simulink model "Model_10_2"  (R2018a)
settings: Solver=VariableStepAuto  StartTime=0.0  StopTime=10.0  RelTol=1e-3
values from neighbouring files (symbols this model uses):
  bias_u = 0.2    [CEE_10.m]    (also in CEE_10_unc.m; CEE_11.m)
  C_I = [1 0 0 0 0]    [CEE_10.m]    (also in CEE_10_performance.m; CEE_11.m)
  covProcess = 100*diag([0.018^2,(0.018*10)^2,0.018^2,(0.018*10)^2,0.025^2])    [CEE_10.m]    (also in CEE_10_performance.m; CEE_10_unc.m; CEE_11.m; CEE_9.m)
  covSensor = ((0.018)^2)*eye(2)    [CEE_10.m]    (also in CEE_10_performance.m = ((2*0.018)^2)*eye(2); CEE_10_unc.m = ((2*0.018)^2)*eye(2); CEE_11.m; CEE_9.m)
  deadzone_u = 2e-1    (= 0.2)    [CEE_10.m]    (also in CEE_10_performance.m; CEE_10_unc.m; CEE_11.m; CEE_9.m = 0.1)
  L = lqe(A, G, C, Qe, Re)    [CEE_10.m]    (also in CEE_10_performance.m; CEE_10_unc.m; CEE_11.m; CEE_9.m)
  pulse = 4    [CEE_10.m]    (also in CEE_10_performance.m; CEE_10_unc.m; CEE_9.m; CEE_9_performance.m)
  saturation_u = 5    [CEE_10.m]    (also in CEE_10_performance.m; CEE_10_unc.m; CEE_11.m; CEE_9.m)
  tc = (1/100)*2*pi/10    (= 0.00628318530718)    [CEE_10.m]    (also in CEE_10_performance.m; CEE_10_unc.m; CEE_11.m; CEE_9.m)
  x0 = [50,0,10,0,0]'*pi/180    [CEE_10.m]    (also in CEE_10_performance.m; CEE_11.m; CEE_9.m; CEE_9_performance.m)
undefined symbols (not defined in the file or in its folder): A, B, C, K
libraries: simulink x2
settings Model: Creator=miguelsilva  LastModifiedBy=leonardopedroso
settings DebuggingCC: LibraryContextMissingDiagnostic=warning
settings SFSimCC: SimUseLocalCustomCode=on
settings RTWCC: RTWUseLocalCustomCode=on

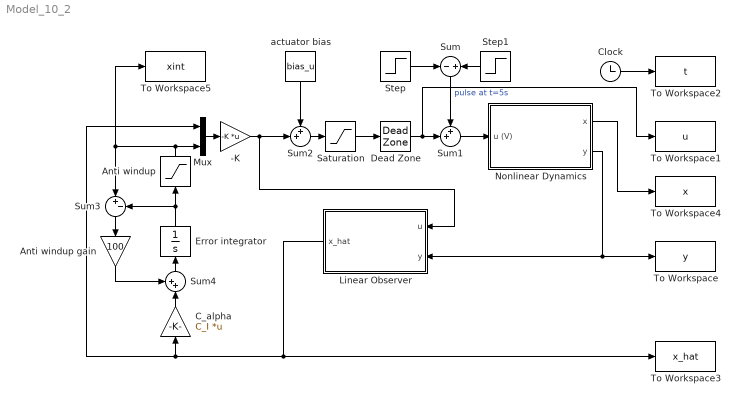
== system Model_10_2 ==
  -K : Gain  Gain=-K  Multiplication=Matrix(K*u) (u vector)
  Anti windup : Saturate  UpperLimit=0.3  LowerLimit=-0.3
  Anti windup gain : Gain  Gain=100
  C_alpha : Gain  Gain=C_I  Multiplication=Matrix(K*u) (u vector)
  Clock : Clock
  "Dead Zone " : DeadZone  LowerValue=-deadzone_u  UpperValue=deadzone_u  SaturateOnIntegerOverflow=on
  Error integrator : Integrator
  "Linear Observer " : Subsystem
  Mux : Mux  Inputs=2
  Nonlinear Dynamics : Subsystem
  "Saturation " : Saturate  UpperLimit=saturation_u  LowerLimit=-saturation_u
  Step : Step  Time=5.1  After=pulse  SampleTime=0
  Step1 : Step  Time=5  After=pulse  SampleTime=0
  Sum : Sum  Inputs=-|+
  Sum1 : Sum  Inputs=++|
  Sum2 : Sum  Inputs=++|
  Sum3 : Sum  Inputs=|+-
  Sum4 : Sum  Inputs=++|
  To Workspace : ToWorkspace  VariableName=y  SampleTime=-1
  To Workspace1 : ToWorkspace  VariableName=u  SampleTime=-1
  To Workspace2 : ToWorkspace  VariableName=t  SampleTime=-1
  To Workspace3 : ToWorkspace  VariableName=x_hat  SampleTime=-1
  To Workspace4 : ToWorkspace  VariableName=x  SampleTime=-1
  To Workspace5 : ToWorkspace  VariableName=xint  SampleTime=-1
  actuator bias : Constant  Value=bias_u
  wires:
  Clock/1 -> To Workspace2/1
  Nonlinear Dynamics/2(y) -> To Workspace/1, "Linear Observer "/2("y ")
  "Linear Observer "/1(x_hat) -> To Workspace3/1, C_alpha/1, Mux/1
  "Saturation "/1 -> "Dead Zone "/1
  Step/1 -> Sum/1
  Step1/1 -> Sum/2
  "Dead Zone "/1 -> To Workspace1/1, Sum1/2
  Sum1/1 -> Nonlinear Dynamics/1(u (V))
  Sum/1 -> Sum1/1  "pulse at t=5s"
  Nonlinear Dynamics/1(x) -> To Workspace4/1
  Mux/1 -> -K/1
  -K/1 -> Sum2/2, "Linear Observer "/1(u)
  Sum2/1 -> "Saturation "/1
  actuator bias/1 -> Sum2/1
  Anti windup/1 -> Sum3/1, To Workspace5/1, Mux/2
  Error integrator/1 -> Sum3/2, Anti windup/1
  Sum4/1 -> Error integrator/1
  C_alpha/1 -> Sum4/2
  Sum3/1 -> Anti windup gain/1
  Anti windup gain/1 -> Sum4/1

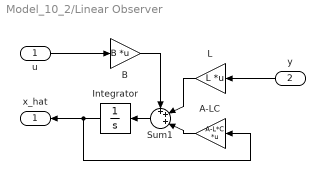
== system Model_10_2/Linear Observer  ==
  u : Inport
  "y " : Inport  Port=2
  A-LC : Gain  Gain=A-L*C  Multiplication=Matrix(K*u) (u vector)
  B : Gain  Gain=B  Multiplication=Matrix(K*u) (u vector)
  Integrator : Integrator  InitialCondition=zeros(5,1)
  L : Gain  Gain=L  Multiplication=Matrix(K*u) (u vector)
  Sum1 : Sum  Inputs=+++|
  x_hat : Outport
  wires:
  Integrator/1 -> x_hat/1, A-LC/1
  L/1 -> Sum1/2
  "y "/1 -> L/1
  Sum1/1 -> Integrator/1
  A-LC/1 -> Sum1/3
  B/1 -> Sum1/1
  u/1 -> B/1

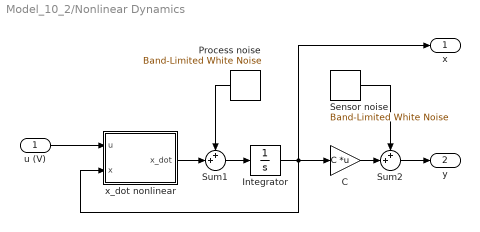
== system Model_10_2/Nonlinear Dynamics ==
  u (V) : Inport
  C : Gain  Gain=C  Multiplication=Matrix(K*u) (u vector)
  Integrator : Integrator  InitialCondition=x0
  Process noise : simulink/Sources/Band-Limited White Noise  Cov=diag(covProcess)*tc  Ts=tc  seed=[23341]
  Sensor noise : simulink/Sources/Band-Limited White Noise  Cov=diag(covSensor)*tc  Ts=tc  seed=[23341]
  Sum1 : Sum  Inputs=++|
  Sum2 : Sum  Inputs=++|
  x_dot nonlinear : MATLAB Function  TreatAsAtomicUnit=on
  x : Outport
  y : Outport  Port=2
  wires:
  Sum2/1 -> y/1
  x_dot nonlinear/1(x_dot) -> Sum1/2
  Process noise/1 -> Sum1/1
  Sum1/1 -> Integrator/1
  Integrator/1 -> C/1, x/1, x_dot nonlinear/2(x)
  Sensor noise/1 -> Sum2/1
  C/1 -> Sum2/2
  u (V)/1 -> x_dot nonlinear/1(u)

== matlab function Model_10_2/Nonlinear Dynamics/x_dot nonlinear ==
  data: u input; x_dot output; x input; NLM parameter
function x_dot = x_dot(u,x,NLM)

x_dot = zeros(5,1);
x_dot(1) = x(2);
x_dot(2) = (-NLM.J2*(NLM.Ka1*x(2)-NLM.Kf*x(5)+...
    x(4)*(NLM.Lcm2*NLM.Le1*NLM.m2*x(4)+2*NLM.J2*x(2)*cos(x(3)))*sin(x(3)))+...
    NLM.Lcm2*NLM.Le1*NLM.m2*cos(x(3))*(-NLM.Ka2*x(4)+(NLM.g*NLM.Lcm2*NLM.m2+NLM.J2*x(2)^2*cos(x(3)))*sin(x(3))))/...
    (-NLM.Lcm2^2*NLM.Le1^2*NLM.m2^2*cos(x(3))^2+NLM.J2*(NLM.J0+NLM.J2*sin(x(3))^2));
x_dot(3) = x(4);
x_dot(4) = (NLM.J0*NLM.Ka2*x(4)-NLM.g*NLM.Lcm2*NLM.m2*sin(x(3))*(NLM.J0+NLM.J2*sin(x(3))^2)+...
    cos(x(3))*((-NLM.J0*NLM.J2*x(2)^2+NLM.Lcm2^2*NLM.Le1^2*NLM.m2^2*x(4)^2)*sin(x(3))-...
    NLM.J2^2*x(2)^2*sin(x(3))^3+NLM.Lcm2*NLM.Le1*NLM.m2*(NLM.Ka1*x(2)-NLM.Kf*x(5)+NLM.J2*x(2)*x(4)*sin(2*x(3)))))/...
    (NLM.Lcm2^2*NLM.Le1^2*NLM.m2^2*cos(x(3))^2-NLM.J2*(NLM.J0+NLM.J2*sin(x(3))^2));
x_dot(5) = (-NLM.Kt*x(2)-NLM.R*x(5)+u(1))/NLM.Lb;
